simulink model "SISO_To_Workspace_Animation"  (R2024a)
settings: Solver=VariableStepAuto  StartTime=0.0  StopTime=10.0  RelTol=1e-3
undefined symbols (not defined in the file or in its folder): DINT, slplc
settings Model: Creator=Jack Vranicar  LastModifiedBy=Jack Vranicar

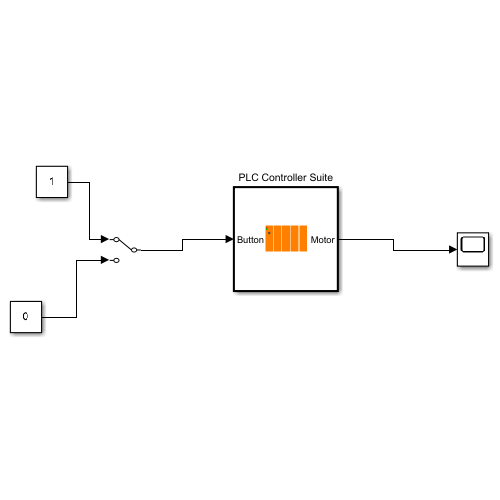
[thumbnail: Simulink's stored preview of the top-level diagram]
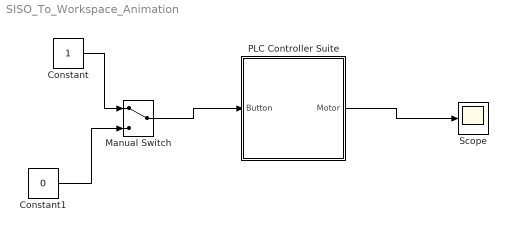
== system SISO_To_Workspace_Animation ==
  Constant : Constant  OutDataTypeStr=boolean
  Constant1 : Constant  Value=0  OutDataTypeStr=boolean
  Manual Switch : ManualSwitch
  PLC Controller Suite : Subsystem  TreatAsAtomicUnit=on  mask{PLCBlockType=PLCController, PLCPOUType=PLC Controller}
      mask init:
      | slplc.callbacks.initController(gcb);
      settings: OpenFcn=slplc.callbacks.openPOUBlock(gcb);
      mask Help: web([docroot '/plccoder/ref/plccontrollersuite' '.html']);
      mask DialogControl PLCBlockTitle Prompt: PLC Controller Block
  Scope : Scope
  wires:
  PLC Controller Suite/1(Motor) -> Scope/1
  Constant/1 -> Manual Switch/1
  Constant1/1 -> Manual Switch/2
  Manual Switch/1 -> PLC Controller Suite/1(Button)

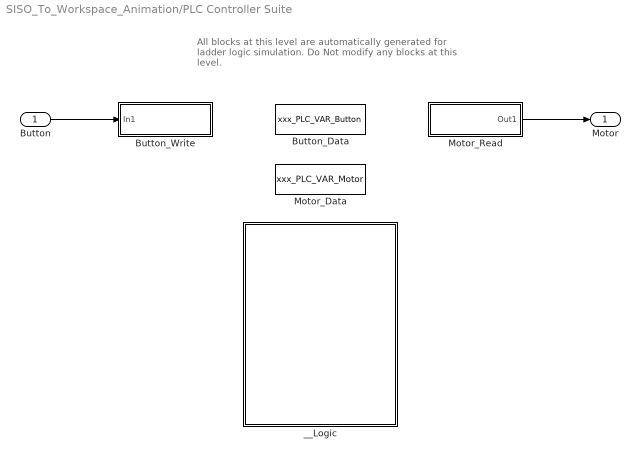
== system SISO_To_Workspace_Animation/PLC Controller Suite ==
  note: All blocks at this level are automatically generated for ladder logic simulation.
      | Do Not modify any blocks at this level.
  Button : Inport  OutDataTypeStr=boolean
  Button_Data : DataStoreMemory  Tag=POUVariable  Priority=10  DataStoreName=xxx_PLC_VAR_Button  ShowAdditionalParam=off  OutDataTypeStr=boolean  Dimensions=1
  Button_Write : Subsystem  Priority=11  DisableCoverage=on  TreatAsAtomicUnit=on  mask{PLCOperandTag=Button, PLCOperandExpression=xxx_PLC_VAR_Button, PLCBlockType=VarWrite, PLCPOUType=VarWrite}
      mask prompts: PLCOperandTag "Operand Tag:"
      mask init:
      | slplc.callbacks.initInstruction(gcb);
      mask Help: web([docroot '/plccoder/ref/varwrite' '.html']);
      mask DialogControl PLCBlockTitle Prompt: Variable Write
      mask Display: disp(get_param(gcb, 'PLCOperandTag'));
  Motor_Data : DataStoreMemory  Tag=POUVariable  Priority=10  DataStoreName=xxx_PLC_VAR_Motor  ShowAdditionalParam=off  OutDataTypeStr=boolean  Dimensions=1
  Motor_Read : Subsystem  Priority=13  DisableCoverage=on  TreatAsAtomicUnit=on  mask{PLCOperandTag=Motor, PLCOperandExpression=xxx_PLC_VAR_Motor, PLCBlockType=VarRead, PLCPOUType=VarRead}
      mask prompts: PLCOperandTag "Operand Tag"
      mask init:
      | block = gcb;
      | maskObj = Simulink.Mask.get(block);
      | maskObj.Display = sprintf('disp(''%s'');', PLCOperandTag);
      | slplc.callbacks.initInstruction(gcb);
      mask Help: web([docroot '/plccoder/ref/varread' '.html']);
      mask DialogControl PLCBlockTitle Prompt: Variable Read
      mask Display: disp('Motor');
  __Logic : Subsystem  Priority=12  TreatAsAtomicUnit=on
  Motor : Outport
  wires:
  Button/1 -> Button_Write/1(In1)
  Motor_Read/1(Out1) -> Motor/1

== system SISO_To_Workspace_Animation/PLC Controller Suite/Button_Write ==
  In1 : Inport
  __CoreVarWrite : Subsystem  Tag=CoreVarWriteBlock  DisableCoverage=on  TreatAsAtomicUnit=on  mask{PLCBlockType=CoreVarWrite}
      mask init:
      | slplc.callbacks.initCoreVariable(gcb, 'write');
      mask DialogControl PLCBlockTitle Prompt: Core Variable Write
  wires:
  In1/1 -> __CoreVarWrite/1(u)

== system SISO_To_Workspace_Animation/PLC Controller Suite/Motor_Read ==
  __CoreVarRead : Subsystem  Tag=CoreVarReadBlock  DisableCoverage=on  TreatAsAtomicUnit=on  mask{PLCBlockType=CoreVarRead}
      mask init:
      | slplc.callbacks.initCoreVariable(gcb, 'read');
      mask DialogControl PLCBlockTitle Prompt: Core Variable Read
  Out1 : Outport  VectorParamsAs1DForOutWhenUnconnected=off
  wires:
  __CoreVarRead/1(y) -> Out1/1

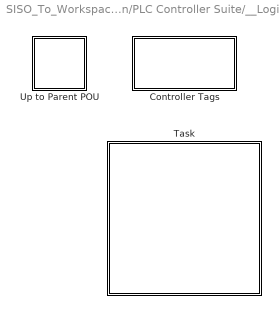
== system SISO_To_Workspace_Animation/PLC Controller Suite/__Logic ==
  Controller Tags : Subsystem  Tag=ControllerVariableSS  DisableCoverage=on  TreatAsAtomicUnit=on  mask{PLCVarButtonName=Button, PLCVarButtonAddress=<empty>, PLCVarButtonMapping=Input Symbol, PLCVarButtonPortIndex=1, PLCVarButtonDataType=boolean, PLCVarButtonSize=1, PLCVarButtonInitialValue=0, PLCVarButtonToDelete=off, PLCVarMotorName=Motor, PLCVarMotorAddress=<empty>, PLCVarMotorMapping=Output Symbol, PLCVarMotorPortIndex=1, PLCVarMotorDataType=boolean, PLCVarMotorSize=1, PLCVarMotorInitialValue=0, PLCVarMotorToDelete=off}
      mask init:
      | slplc.callbacks.initControllerVarSS(gcb);
      settings: OpenFcn=slplc.callbacks.openControllerVariableSS(gcb);
      mask Help: web([docroot '/plccoder/ref/controllertags' '.html']);
      mask TypeOptions PLCVarButtonMapping: Global Variable | Input Symbol | Output Symbol
      mask Callback PLCVarButtonMapping: slplc.callbacks.updateControllerVarSS(gcb);
      mask TypeOptions PLCVarButtonPortIndex: 1 | 2
      mask TypeOptions PLCVarMotorMapping: Global Variable | Input Symbol | Output Symbol
      mask Callback PLCVarMotorMapping: slplc.callbacks.updateControllerVarSS(gcb);
      mask TypeOptions PLCVarMotorPortIndex: 1 | 2
      mask DialogControl PLCBlockTitle Prompt: Global Variable and Symbol Spreadsheet
      mask DialogControl PLCVarListHeaderName Prompt: Name
      mask DialogControl PLCVarListHeaderAddress Prompt: Address (At)
      mask DialogControl PLCVarListHeaderMapping Prompt: Mapping Type
      mask DialogControl PLCVarListHeaderPortIndex Prompt: Port
      mask DialogControl PLCVarListHeaderDataType Prompt: Data Type
      mask DialogControl PLCVarListHeaderSize Prompt: Size
      mask DialogControl PLCVarListHeaderInitialValue Prompt: Initial Value
      mask DialogControl PLCVarListHeaderToDelete Prompt: Delete
  Task : Subsystem  TreatAsAtomicUnit=on  mask{PLCBlockType=Task, PLCPOUType=Task, PLCTaskWatchDog=0}
      settings: OpenFcn=slplc.callbacks.openTaskBlock(gcb);
      mask Help: web([docroot '/plccoder/ref/task' '.html']);
      mask DialogControl PLCBlockTitle Prompt: Task
  Up to Parent POU : Subsystem  DisableCoverage=on  TreatAsAtomicUnit=on  mask{PLCBlockType=OpenParentPOU}
      settings: OpenFcn=slplc.callbacks.openParentPOUBlock(gcb);
      mask Help: web([docroot '/plccoder/ref/uptoparentpou' '.html']);
      mask DialogControl PLCBlockTitle Prompt: Add Single Rung

== system SISO_To_Workspace_Animation/PLC Controller Suite/Button_Write/__CoreVarWrite ==
  u : Inport
  DataWrite : DataStoreWrite  DataStoreName=xxx_PLC_VAR_Button  IndexOptions=Index vector (dialog)  Indices=1  OutputSizes=1
  wires:
  u/1 -> DataWrite/1

== system SISO_To_Workspace_Animation/PLC Controller Suite/Motor_Read/__CoreVarRead ==
  DataRead : DataStoreRead  DataStoreName=xxx_PLC_VAR_Motor  IndexOptions=Index vector (dialog)  Indices=1  OutputSizes=1
  y : Outport  VectorParamsAs1DForOutWhenUnconnected=off
  wires:
  DataRead/1 -> y/1

== system SISO_To_Workspace_Animation/PLC Controller Suite/__Logic/Controller Tags ==

== system SISO_To_Workspace_Animation/PLC Controller Suite/__Logic/Task ==
  Program : Subsystem  TreatAsAtomicUnit=on  mask{PLCPOUType=Program, PLCPOULanguage=LD, PLCBlockType=LDProgram}
      mask prompts: PLCPOUType "POU Type:"
      mask init:
      | slplc.callbacks.initProgram(gcb);
      settings: OpenFcn=slplc.callbacks.openPOUBlock(gcb);
      mask Help: web([docroot '/plccoder/ref/ldprogram' '.html']);
      mask DialogControl PLCBlockTitle Prompt: Program
      mask DialogControl PLCEditPOU Prompt: Edit POU
      mask DialogControl PLCEditInterface Prompt: Edit Variables
  Up to Parent POU : Subsystem  DisableCoverage=on  TreatAsAtomicUnit=on  mask{PLCBlockType=OpenParentPOU}
      settings: OpenFcn=slplc.callbacks.openParentPOUBlock(gcb);
      mask Help: web([docroot '/plccoder/ref/uptoparentpou' '.html']);
      mask DialogControl PLCBlockTitle Prompt: Add Single Rung

== system SISO_To_Workspace_Animation/PLC Controller Suite/__Logic/Up to Parent POU ==

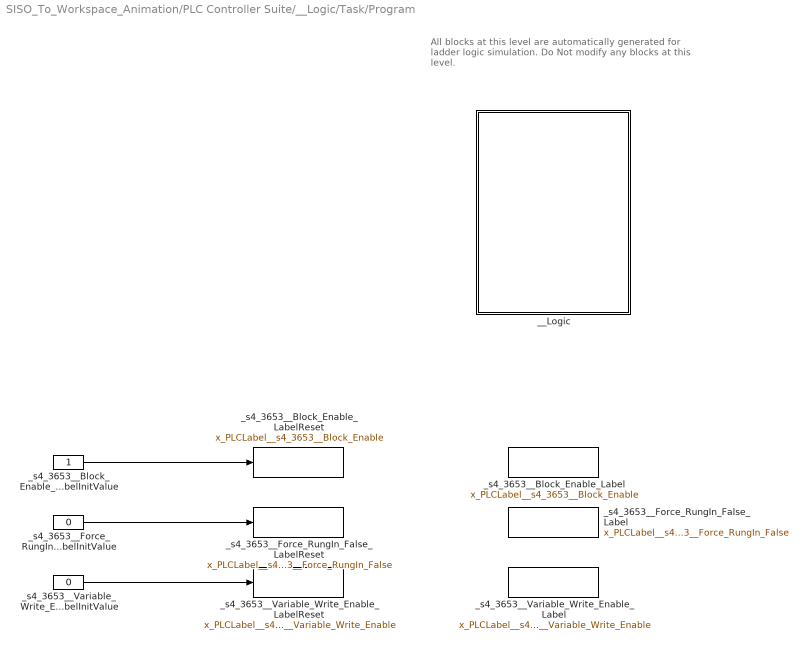
== system SISO_To_Workspace_Animation/PLC Controller Suite/__Logic/Task/Program ==
  note: All blocks at this level are automatically generated for ladder logic simulation.
      | Do Not modify any blocks at this level.
  __Logic : Subsystem  Priority=12  TreatAsAtomicUnit=on
  _s4_3653__Block_Enable_Label : DataStoreMemory  Priority=10  DataStoreName=x_PLCLabel__s4_3653__Block_Enable  InitialValue=1  ShowAdditionalParam=off  OutDataTypeStr=BOOL  Dimensions=1
  _s4_3653__Block_Enable_LabelInitValue : Constant  OutDataTypeStr=BOOL
  _s4_3653__Block_Enable_LabelReset : DataStoreWrite  Priority=11  DataStoreName=x_PLCLabel__s4_3653__Block_Enable  IndexOptions=Index vector (dialog)  Indices=1  OutputSizes=1
  _s4_3653__Force_RungIn_False_Label : DataStoreMemory  Priority=10  DataStoreName=x_PLCLabel__s4_3653__Force_RungIn_False  ShowAdditionalParam=off  OutDataTypeStr=BOOL  Dimensions=1
  _s4_3653__Force_RungIn_False_LabelInitValue : Constant  Value=0  OutDataTypeStr=BOOL
  _s4_3653__Force_RungIn_False_LabelReset : DataStoreWrite  Priority=11  DataStoreName=x_PLCLabel__s4_3653__Force_RungIn_False  IndexOptions=Index vector (dialog)  Indices=1  OutputSizes=1
  _s4_3653__Variable_Write_Enable_Label : DataStoreMemory  Priority=10  DataStoreName=x_PLCLabel__s4_3653__Variable_Write_Enable  ShowAdditionalParam=off  OutDataTypeStr=BOOL  Dimensions=1
  _s4_3653__Variable_Write_Enable_LabelInitValue : Constant  Value=0  OutDataTypeStr=BOOL
  _s4_3653__Variable_Write_Enable_LabelReset : DataStoreWrite  Priority=11  DataStoreName=x_PLCLabel__s4_3653__Variable_Write_Enable  IndexOptions=Index vector (dialog)  Indices=1  OutputSizes=1
  wires:
  _s4_3653__Block_Enable_LabelInitValue/1 -> _s4_3653__Block_Enable_LabelReset/1
  _s4_3653__Variable_Write_Enable_LabelInitValue/1 -> _s4_3653__Variable_Write_Enable_LabelReset/1
  _s4_3653__Force_RungIn_False_LabelInitValue/1 -> _s4_3653__Force_RungIn_False_LabelReset/1

== system SISO_To_Workspace_Animation/PLC Controller Suite/__Logic/Task/Up to Parent POU ==

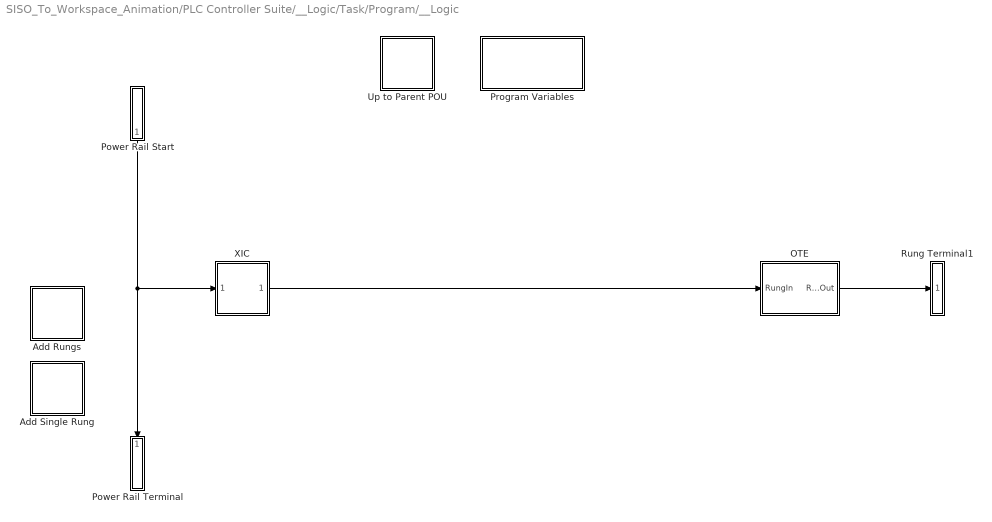
== system SISO_To_Workspace_Animation/PLC Controller Suite/__Logic/Task/Program/__Logic ==
  Add Rungs : Subsystem  DisableCoverage=on  TreatAsAtomicUnit=on  mask{PLCRungNumberToAdd=2, PLCBlockType=AddRungs}
      mask prompts: PLCRungNumberToAdd "Rung Number:"
      mask Help: web([docroot '/plccoder/ref/addrungs' '.html']);
      mask DialogControl PLCAddRungs Prompt: Add Rungs
      mask DialogControl PLCRungAddButton Prompt: Add
      mask DialogControl PLCRungAddButton Callback: slplc.callbacks.addLadderRungs(gcb);
      mask Display: disp(sprintf(['Add' newline 'Rungs']));
  Add Single Rung : Subsystem  DisableCoverage=on  TreatAsAtomicUnit=on  mask{PLCRungNumberToAdd=1, PLCBlockType=AddSingleRung}
      settings: OpenFcn=slplc.callbacks.addLadderRungs(gcb);
      mask Help: web([docroot '/plccoder/ref/addsinglerung' '.html']);
      mask DialogControl PLCAddRung Prompt: Add Single Rung
      mask Display: disp(sprintf(['Add' newline '1 Rung']));
  OTE : Subsystem  Priority=3  TreatAsAtomicUnit=on  mask{PLCOperandTag=Motor, PLCBlockType=OTE, PLCPOUType=Coil, PLCOperandExpression=xxx_PLC_VAR_Motor}
      mask prompts: PLCOperandTag "Operand Tag:"
      mask init:
      | slplc.callbacks.initInstruction(gcb);
      settings: AttributesFormatString=%<PLCOperandTag>
      mask Help: web([docroot '/plccoder/ref/ote' '.html']);
      mask DialogControl PLCBlockTitle Prompt: Output Energize (OTE)
  Power Rail Start : Subsystem  Priority=1  DisableCoverage=on  TreatAsAtomicUnit=on  mask{PLCBlockType=PowerRailStart}
      mask Help: web([docroot '/plccoder/ref/powerrailstart' '.html']);
      mask DialogControl PLCBlockTitle Prompt: Power Rail Start
      mask DialogControl PLCBlockDesc Prompt: This is the ladder diagram left power rail start block.
  Power Rail Terminal : Subsystem  DisableCoverage=on  TreatAsAtomicUnit=on  mask{PLCBlockType=PowerRailTerminal}
      mask Help: web([docroot '/plccoder/ref/powerrailterminal' '.html']);
      mask DialogControl PLCBlockTitle Prompt: Power Rail Terminal
      mask DialogControl PLCBlockDesc Prompt: This is the ladder diagram left power rail terminal block.
  Program Variables : Subsystem  Tag=ProgramVariableSS  DisableCoverage=on  TreatAsAtomicUnit=on  mask{PLCVarButtonName=Button, PLCVarButtonScope=External, PLCVarButtonPortType=Hidden, PLCVarButtonPortIndex=2, PLCVarButtonDataType=DINT, PLCVarButtonSize=-1, PLCVarButtonInitialValue=0, PLCVarButtonToDelete=off, PLCVarMotorName=Motor, PLCVarMotorScope=External, PLCVarMotorPortType=Hidden, PLCVarMotorPortIndex=2, PLCVarMotorDataType=DINT, PLCVarMotorSize=-1, PLCVarMotorInitialValue=0, PLCVarMotorToDelete=off}
      mask init:
      | slplc.callbacks.initPOUVarSS(gcb);
      settings: OpenFcn=slplc.callbacks.openProgramVariableSS(gcb);
      mask Help: web([docroot '/plccoder/ref/programvariables' '.html']);
      mask TypeOptions PLCVarButtonScope: Local | External
      mask Callback PLCVarButtonScope: slplc.callbacks.updatePOUVarSS(gcb);
      mask TypeOptions PLCVarButtonPortType: Hidden | Inport | Outport
      mask Callback PLCVarButtonPortType: slplc.callbacks.updatePOUVarSS(gcb);
      mask TypeOptions PLCVarButtonPortIndex: 1 | 2
      mask TypeOptions PLCVarMotorScope: Local | External
      mask Callback PLCVarMotorScope: slplc.callbacks.updatePOUVarSS(gcb);
      mask TypeOptions PLCVarMotorPortType: Hidden | Inport | Outport
      mask Callback PLCVarMotorPortType: slplc.callbacks.updatePOUVarSS(gcb);
      mask TypeOptions PLCVarMotorPortIndex: 1 | 2
      mask DialogControl PLCBlockTitle Prompt: Program Variable Spreadsheet
      mask DialogControl PLCVarListHeaderName Prompt: Name
      mask DialogControl PLCVarListHeaderScope Prompt: Scope
      mask DialogControl PLCVarListHeaderDataType Prompt: Data Type
      mask DialogControl PLCVarListHeaderSize Prompt: Size
      mask DialogControl PLCVarListHeaderInitialValue Prompt: Initial Value
      mask DialogControl PLCVarListHeaderToDelete Prompt: Delete
  Rung Terminal1 : Subsystem  Priority=4  DisableCoverage=on  TreatAsAtomicUnit=on  mask{PLCRungTerminalIndex=1, PLCBlockType=RungTerminal}
      settings: AttributesFormatString=Rung %<PLCRungTerminalIndex>
      mask Help: web([docroot '/plccoder/ref/rungterminal' '.html']);
      mask DialogControl PLCBlockTitle Prompt: Rung Terminal
      mask DialogControl PLCBlockDescText Prompt: This is the ladder diagram rung terminal.
  Up to Parent POU : Subsystem  DisableCoverage=on  TreatAsAtomicUnit=on  mask{PLCBlockType=OpenParentPOU}
      settings: OpenFcn=slplc.callbacks.openParentPOUBlock(gcb);
      mask Help: web([docroot '/plccoder/ref/uptoparentpou' '.html']);
      mask DialogControl PLCBlockTitle Prompt: Add Single Rung
  XIC : Subsystem  Priority=2  TreatAsAtomicUnit=on  mask{PLCOperandTag=Button, PLCBlockType=XIC, PLCPOUType=Contact, PLCOperandExpression=xxx_PLC_VAR_Button}
      mask prompts: PLCOperandTag "Operand Tag:"
      mask init:
      | slplc.callbacks.initInstruction(gcb);
      settings: AttributesFormatString=%<PLCOperandTag>
      mask Help: web([docroot '/plccoder/ref/xic' '.html']);
      mask DialogControl PLCBlockTitle Prompt: Examine If Closed (XIC)
  wires:
  Power Rail Start/1(PowerOut) -> Power Rail Terminal/1(PowerIn), XIC/1(RungIn)
  XIC/1(RungOut) -> OTE/1(RungIn)
  OTE/1(RungOut) -> Rung Terminal1/1(RungIn)

== system SISO_To_Workspace_Animation/PLC Controller Suite/__Logic/Task/Program/__Logic/Add Rungs ==

== system SISO_To_Workspace_Animation/PLC Controller Suite/__Logic/Task/Program/__Logic/Add Single Rung ==

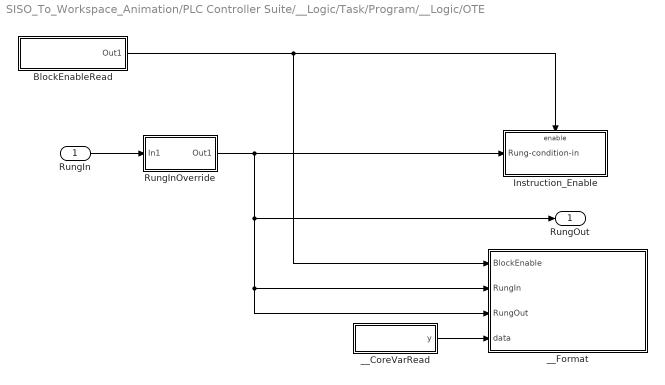
== system SISO_To_Workspace_Animation/PLC Controller Suite/__Logic/Task/Program/__Logic/OTE ==
  RungIn : Inport  PortDimensions=1
  BlockEnableRead : Subsystem  DisableCoverage=on  TreatAsAtomicUnit=on  mask{PLCLabelTag=_Block_Enable, PLCBlockType=BlockEnableRead}
      mask prompts: PLCLabelTag "Label Tag:"
      mask init:
      | block = gcb;
      | maskObj = Simulink.Mask.get(block);
      | maskObj.Display = sprintf('disp(''%s'');', PLCLabelTag);
      mask Help: web([docroot '/plccoder/ref/blockenableread' '.html']);
      mask DialogControl PLCBlockTitle Prompt: Block Enable Read
      mask Display: disp('_Block_Enable');
  Instruction_Enable : Subsystem  Priority=12  TreatAsAtomicUnit=on
  RungInOverride : Subsystem  DisableCoverage=on  TreatAsAtomicUnit=on
  __CoreVarRead : Subsystem  Tag=CoreVarReadBlock  DisableCoverage=on  TreatAsAtomicUnit=on  mask{PLCBlockType=CoreVarRead}
      mask init:
      | slplc.callbacks.initCoreVariable(gcb, 'read');
      mask Help: web([docroot '/plccoder/ref/__corevarread' '.html']);
      mask DialogControl PLCBlockTitle Prompt: Core Variable Read
  __Format : MATLAB Function  Tag=PLC_Format_Boolean  Priority=20  DisableCoverage=on  InitFcn=slplc.utils.setBlockAppearance('reset', '%<PLCOperandTag>');  StopFcn=slplc.utils.setBlockAppearance('reset', '%<PLCOperandTag>');  TreatAsAtomicUnit=on
  RungOut : Outport  OutDataTypeStr=BOOL  PortDimensions=1  InitialOutput=false  VectorParamsAs1DForOutWhenUnconnected=off
  wires:
  RungIn/1 -> RungInOverride/1(In1)
  BlockEnableRead/1(Out1) -> __Format/1(BlockEnable), Instruction_Enable/Enable
  RungInOverride/1(Out1) -> __Format/2(RungIn), __Format/3(RungOut), RungOut/1, Instruction_Enable/1(Rung-condition-in)
  __CoreVarRead/1(y) -> __Format/4(data)

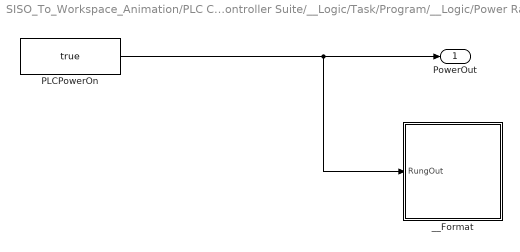
== system SISO_To_Workspace_Animation/PLC Controller Suite/__Logic/Task/Program/__Logic/Power Rail Start ==
  PLCPowerOn : Constant  Value=true  OutDataTypeStr=BOOL
  __Format : MATLAB Function  Tag=PLC_Format_ENO  Priority=20  DisableCoverage=on  InitFcn=slplc.utils.setBlockAppearance('reset', '', {'black', 'black'});  StopFcn=slplc.utils.setBlockAppearance('reset', '', {'black', 'black'});  TreatAsAtomicUnit=on
  PowerOut : Outport  VectorParamsAs1DForOutWhenUnconnected=off
  wires:
  PLCPowerOn/1 -> __Format/1(RungOut), PowerOut/1

== system SISO_To_Workspace_Animation/PLC Controller Suite/__Logic/Task/Program/__Logic/Power Rail Terminal ==
  PowerIn : Inport
  Terminator3 : Terminator
  wires:
  PowerIn/1 -> Terminator3/1

== system SISO_To_Workspace_Animation/PLC Controller Suite/__Logic/Task/Program/__Logic/Program Variables ==

== system SISO_To_Workspace_Animation/PLC Controller Suite/__Logic/Task/Program/__Logic/Rung Terminal1 ==
  RungIn : Inport
  Terminator : Terminator
  wires:
  RungIn/1 -> Terminator/1

== system SISO_To_Workspace_Animation/PLC Controller Suite/__Logic/Task/Program/__Logic/Up to Parent POU ==

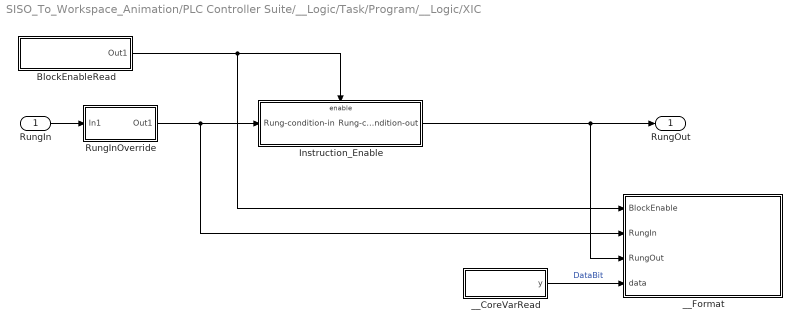
== system SISO_To_Workspace_Animation/PLC Controller Suite/__Logic/Task/Program/__Logic/XIC ==
  RungIn : Inport  PortDimensions=1
  BlockEnableRead : Subsystem  DisableCoverage=on  TreatAsAtomicUnit=on  mask{PLCLabelTag=_Block_Enable, PLCBlockType=BlockEnableRead}
      mask prompts: PLCLabelTag "Label Tag:"
      mask init:
      | block = gcb;
      | maskObj = Simulink.Mask.get(block);
      | maskObj.Display = sprintf('disp(''%s'');', PLCLabelTag);
      mask Help: web([docroot '/plccoder/ref/blockenableread' '.html']);
      mask DialogControl PLCBlockTitle Prompt: Block Enable Read
      mask Display: disp('_Block_Enable');
  Instruction_Enable : Subsystem  Priority=12  TreatAsAtomicUnit=on
  RungInOverride : Subsystem  DisableCoverage=on  TreatAsAtomicUnit=on
  __CoreVarRead : Subsystem  Tag=CoreVarReadBlock  DisableCoverage=on  TreatAsAtomicUnit=on  mask{PLCBlockType=CoreVarRead}
      mask init:
      | slplc.callbacks.initCoreVariable(gcb, 'read');
      mask Help: web([docroot '/plccoder/ref/__corevarread' '.html']);
      mask DialogControl PLCBlockTitle Prompt: Core Variable Read
  __Format : MATLAB Function  Tag=PLC_Format_Boolean  Priority=20  DisableCoverage=on  InitFcn=slplc.utils.setBlockAppearance('reset', '%<PLCOperandTag>');  StopFcn=slplc.utils.setBlockAppearance('reset', '%<PLCOperandTag>');  TreatAsAtomicUnit=on
  RungOut : Outport  OutDataTypeStr=BOOL  PortDimensions=1  InitialOutput=false  VectorParamsAs1DForOutWhenUnconnected=off
  wires:
  __CoreVarRead/1(y) -> __Format/4(data)  "DataBit"
  RungInOverride/1(Out1) -> Instruction_Enable/1(Rung-condition-in), __Format/2(RungIn)
  BlockEnableRead/1(Out1) -> Instruction_Enable/Enable, __Format/1(BlockEnable)
  Instruction_Enable/1(Rung-condition-out) -> RungOut/1, __Format/3(RungOut)
  RungIn/1 -> RungInOverride/1(In1)

== system SISO_To_Workspace_Animation/PLC Controller Suite/__Logic/Task/Program/__Logic/OTE/BlockEnableRead ==
  __CoreLabelRead : Subsystem  Tag=CoreVarReadBlock  DisableCoverage=on  TreatAsAtomicUnit=on  mask{PLCBlockType=CoreLabelRead}
      mask init:
      | slplc.callbacks.initRoutineLabelRead(gcb);
      mask Help: web([docroot '/plccoder/ref/__corelabelread' '.html']);
      mask DialogControl PLCBlockTitle Prompt: Core Label Read
  Out1 : Outport  VectorParamsAs1DForOutWhenUnconnected=off
  wires:
  __CoreLabelRead/1(Out1) -> Out1/1

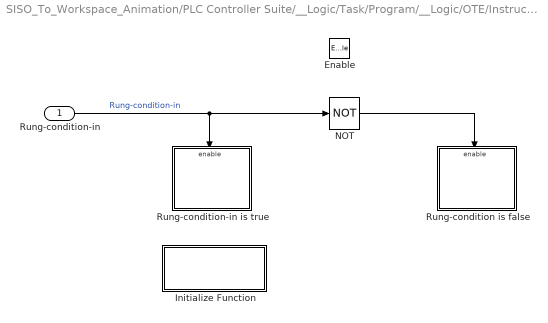
== system SISO_To_Workspace_Animation/PLC Controller Suite/__Logic/Task/Program/__Logic/OTE/Instruction_Enable ==
  Rung-condition-in : Inport  OutDataTypeStr=BOOL
  Enable : EnablePort
  Initialize Function : Subsystem  TreatAsAtomicUnit=on
  NOT : Logic  Operator=NOT  IconShape=distinctive  AllPortsSameDT=off  OutDataTypeStr=boolean
  Rung-condition is false : Subsystem  Priority=12  DisableCoverage=on
  Rung-condition-in is true : Subsystem  Priority=12  DisableCoverage=on
  wires:
  NOT/1 -> Rung-condition is false/Enable
  Rung-condition-in/1 -> Rung-condition-in is true/Enable, NOT/1  "Rung-condition-in"

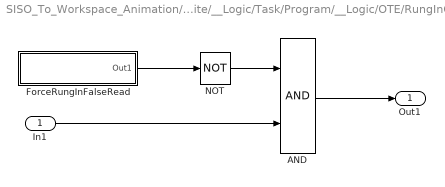
== system SISO_To_Workspace_Animation/PLC Controller Suite/__Logic/Task/Program/__Logic/OTE/RungInOverride ==
  In1 : Inport
  AND : Logic  AllPortsSameDT=off  OutDataTypeStr=boolean
  ForceRungInFalseRead : Subsystem  DisableCoverage=on  TreatAsAtomicUnit=on  mask{PLCLabelTag=_Force_RungIn_False, PLCBlockType=ForceRungInFalseRead}
      mask prompts: PLCLabelTag "Label Tag:"
      mask init:
      | block = gcb;
      | maskObj = Simulink.Mask.get(block);
      | maskObj.Display = sprintf('disp(''%s'');', PLCLabelTag);
      mask Help: web([docroot '/plccoder/ref/forcerunginfalseread' '.html']);
      mask DialogControl PLCBlockTitle Prompt: Force Rung-In False Read
      mask Display: disp('_Force_RungIn_False');
  NOT : Logic  Operator=NOT  IconShape=distinctive  AllPortsSameDT=off  OutDataTypeStr=boolean
  Out1 : Outport  VectorParamsAs1DForOutWhenUnconnected=off
  wires:
  AND/1 -> Out1/1
  In1/1 -> AND/2
  ForceRungInFalseRead/1(Out1) -> NOT/1
  NOT/1 -> AND/1

== system SISO_To_Workspace_Animation/PLC Controller Suite/__Logic/Task/Program/__Logic/OTE/__CoreVarRead ==
  DataRead : DataStoreRead  DataStoreName=xxx_PLC_VAR_Motor  IndexOptions=Index vector (dialog)  Indices=1  OutputSizes=1
  y : Outport  VectorParamsAs1DForOutWhenUnconnected=off
  wires:
  DataRead/1 -> y/1

== system SISO_To_Workspace_Animation/PLC Controller Suite/__Logic/Task/Program/__Logic/XIC/BlockEnableRead ==
  __CoreLabelRead : Subsystem  Tag=CoreVarReadBlock  DisableCoverage=on  TreatAsAtomicUnit=on  mask{PLCBlockType=CoreLabelRead}
      mask init:
      | slplc.callbacks.initRoutineLabelRead(gcb);
      mask Help: web([docroot '/plccoder/ref/__corelabelread' '.html']);
      mask DialogControl PLCBlockTitle Prompt: Core Label Read
  Out1 : Outport  VectorParamsAs1DForOutWhenUnconnected=off
  wires:
  __CoreLabelRead/1(Out1) -> Out1/1

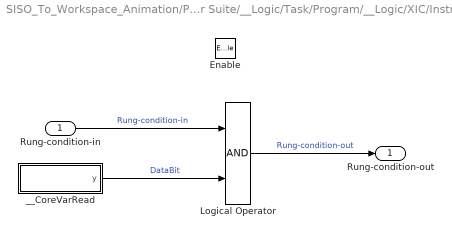
== system SISO_To_Workspace_Animation/PLC Controller Suite/__Logic/Task/Program/__Logic/XIC/Instruction_Enable ==
  Rung-condition-in : Inport  OutDataTypeStr=BOOL
  Enable : EnablePort
  Logical Operator : Logic  OutDataTypeStr=BOOL
  __CoreVarRead : Subsystem  Tag=CoreVarReadBlock  DisableCoverage=on  TreatAsAtomicUnit=on  mask{PLCBlockType=CoreVarRead}
      mask init:
      | slplc.callbacks.initCoreVariable(gcb, 'read');
      mask Help: web([docroot '/plccoder/ref/__corevarread' '.html']);
      mask DialogControl PLCBlockTitle Prompt: Core Variable Read
  Rung-condition-out : Outport  VectorParamsAs1DForOutWhenUnconnected=off
  wires:
  Rung-condition-in/1 -> Logical Operator/1  "Rung-condition-in"
  Logical Operator/1 -> Rung-condition-out/1  "Rung-condition-out"
  __CoreVarRead/1(y) -> Logical Operator/2  "DataBit"

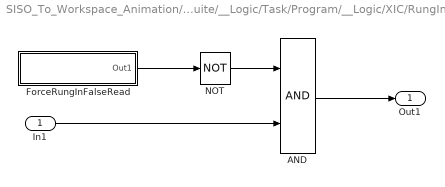
== system SISO_To_Workspace_Animation/PLC Controller Suite/__Logic/Task/Program/__Logic/XIC/RungInOverride ==
  In1 : Inport
  AND : Logic  AllPortsSameDT=off  OutDataTypeStr=boolean
  ForceRungInFalseRead : Subsystem  DisableCoverage=on  TreatAsAtomicUnit=on  mask{PLCLabelTag=_Force_RungIn_False, PLCBlockType=ForceRungInFalseRead}
      mask prompts: PLCLabelTag "Label Tag:"
      mask init:
      | block = gcb;
      | maskObj = Simulink.Mask.get(block);
      | maskObj.Display = sprintf('disp(''%s'');', PLCLabelTag);
      mask Help: web([docroot '/plccoder/ref/forcerunginfalseread' '.html']);
      mask DialogControl PLCBlockTitle Prompt: Force Rung-In False Read
      mask Display: disp('_Force_RungIn_False');
  NOT : Logic  Operator=NOT  IconShape=distinctive  AllPortsSameDT=off  OutDataTypeStr=boolean
  Out1 : Outport  VectorParamsAs1DForOutWhenUnconnected=off
  wires:
  AND/1 -> Out1/1
  In1/1 -> AND/2
  ForceRungInFalseRead/1(Out1) -> NOT/1
  NOT/1 -> AND/1

== system SISO_To_Workspace_Animation/PLC Controller Suite/__Logic/Task/Program/__Logic/XIC/__CoreVarRead ==
  DataRead : DataStoreRead  DataStoreName=xxx_PLC_VAR_Button  IndexOptions=Index vector (dialog)  Indices=1  OutputSizes=1
  y : Outport  VectorParamsAs1DForOutWhenUnconnected=off
  wires:
  DataRead/1 -> y/1

== system SISO_To_Workspace_Animation/PLC Controller Suite/__Logic/Task/Program/__Logic/OTE/BlockEnableRead/__CoreLabelRead ==
  DataRead : DataStoreRead  DataStoreName=x_PLCLabel__s4_3653__Block_Enable  IndexOptions=Index vector (dialog)  Indices=1  OutputSizes=1
  Out1 : Outport  VectorParamsAs1DForOutWhenUnconnected=off
  wires:
  DataRead/1 -> Out1/1

== system SISO_To_Workspace_Animation/PLC Controller Suite/__Logic/Task/Program/__Logic/OTE/Instruction_Enable/Initialize Function ==
  Constant : Constant  Value=0  OutDataTypeStr=BOOL
  Event Listener : EventListener  DisableCoverage=on  EventName=reset
  __CoreVarWrite : Subsystem  Tag=CoreVarWriteBlock  DisableCoverage=on  TreatAsAtomicUnit=on  mask{PLCBlockType=CoreVarWrite}
      mask init:
      | slplc.callbacks.initCoreVariable(gcb, 'write');
      mask Help: web([docroot '/plccoder/ref/__corevarwrite' '.html']);
      mask DialogControl PLCBlockTitle Prompt: Core Variable Write
  wires:
  Constant/1 -> __CoreVarWrite/1(u)

== system SISO_To_Workspace_Animation/PLC Controller Suite/__Logic/Task/Program/__Logic/OTE/Instruction_Enable/Rung-condition is false ==
  Enable : EnablePort
  Constant : Constant  Value=0  OutDataTypeStr=BOOL
  __CoreVarWrite : Subsystem  Tag=CoreVarWriteBlock  DisableCoverage=on  TreatAsAtomicUnit=on  mask{PLCBlockType=CoreVarWrite}
      mask init:
      | slplc.callbacks.initCoreVariable(gcb, 'write');
      mask Help: web([docroot '/plccoder/ref/__corevarwrite' '.html']);
      mask DialogControl PLCBlockTitle Prompt: Core Variable Write
  wires:
  Constant/1 -> __CoreVarWrite/1(u)

== system SISO_To_Workspace_Animation/PLC Controller Suite/__Logic/Task/Program/__Logic/OTE/Instruction_Enable/Rung-condition-in is true ==
  Enable : EnablePort
  Constant : Constant  OutDataTypeStr=BOOL
  __CoreVarWrite : Subsystem  Tag=CoreVarWriteBlock  DisableCoverage=on  TreatAsAtomicUnit=on  mask{PLCBlockType=CoreVarWrite}
      mask init:
      | slplc.callbacks.initCoreVariable(gcb, 'write');
      mask Help: web([docroot '/plccoder/ref/__corevarwrite' '.html']);
      mask DialogControl PLCBlockTitle Prompt: Core Variable Write
  wires:
  Constant/1 -> __CoreVarWrite/1(u)

== system SISO_To_Workspace_Animation/PLC Controller Suite/__Logic/Task/Program/__Logic/OTE/RungInOverride/ForceRungInFalseRead ==
  __CoreLabelRead : Subsystem  Tag=CoreVarReadBlock  DisableCoverage=on  TreatAsAtomicUnit=on  mask{PLCBlockType=CoreLabelRead}
      mask init:
      | slplc.callbacks.initRoutineLabelRead(gcb);
      mask Help: web([docroot '/plccoder/ref/__corelabelread' '.html']);
      mask DialogControl PLCBlockTitle Prompt: Core Label Read
  Out1 : Outport  VectorParamsAs1DForOutWhenUnconnected=off
  wires:
  __CoreLabelRead/1(Out1) -> Out1/1

== system SISO_To_Workspace_Animation/PLC Controller Suite/__Logic/Task/Program/__Logic/XIC/BlockEnableRead/__CoreLabelRead ==
  DataRead : DataStoreRead  DataStoreName=x_PLCLabel__s4_3653__Block_Enable  IndexOptions=Index vector (dialog)  Indices=1  OutputSizes=1
  Out1 : Outport  VectorParamsAs1DForOutWhenUnconnected=off
  wires:
  DataRead/1 -> Out1/1

== system SISO_To_Workspace_Animation/PLC Controller Suite/__Logic/Task/Program/__Logic/XIC/Instruction_Enable/__CoreVarRead ==
  DataRead : DataStoreRead  DataStoreName=xxx_PLC_VAR_Button  IndexOptions=Index vector (dialog)  Indices=1  OutputSizes=1
  y : Outport  VectorParamsAs1DForOutWhenUnconnected=off
  wires:
  DataRead/1 -> y/1

== system SISO_To_Workspace_Animation/PLC Controller Suite/__Logic/Task/Program/__Logic/XIC/RungInOverride/ForceRungInFalseRead ==
  __CoreLabelRead : Subsystem  Tag=CoreVarReadBlock  DisableCoverage=on  TreatAsAtomicUnit=on  mask{PLCBlockType=CoreLabelRead}
      mask init:
      | slplc.callbacks.initRoutineLabelRead(gcb);
      mask Help: web([docroot '/plccoder/ref/__corelabelread' '.html']);
      mask DialogControl PLCBlockTitle Prompt: Core Label Read
  Out1 : Outport  VectorParamsAs1DForOutWhenUnconnected=off
  wires:
  __CoreLabelRead/1(Out1) -> Out1/1

== system SISO_To_Workspace_Animation/PLC Controller Suite/__Logic/Task/Program/__Logic/OTE/Instruction_Enable/Initialize Function/__CoreVarWrite ==
  u : Inport
  DataWrite : DataStoreWrite  DataStoreName=xxx_PLC_VAR_Motor  IndexOptions=Index vector (dialog)  Indices=1  OutputSizes=1
  wires:
  u/1 -> DataWrite/1

== system SISO_To_Workspace_Animation/PLC Controller Suite/__Logic/Task/Program/__Logic/OTE/Instruction_Enable/Rung-condition is false/__CoreVarWrite ==
  u : Inport
  DataWrite : DataStoreWrite  DataStoreName=xxx_PLC_VAR_Motor  IndexOptions=Index vector (dialog)  Indices=1  OutputSizes=1
  wires:
  u/1 -> DataWrite/1

== system SISO_To_Workspace_Animation/PLC Controller Suite/__Logic/Task/Program/__Logic/OTE/Instruction_Enable/Rung-condition-in is true/__CoreVarWrite ==
  u : Inport
  DataWrite : DataStoreWrite  DataStoreName=xxx_PLC_VAR_Motor  IndexOptions=Index vector (dialog)  Indices=1  OutputSizes=1
  wires:
  u/1 -> DataWrite/1

== system SISO_To_Workspace_Animation/PLC Controller Suite/__Logic/Task/Program/__Logic/OTE/RungInOverride/ForceRungInFalseRead/__CoreLabelRead ==
  DataRead : DataStoreRead  DataStoreName=x_PLCLabel__s4_3653__Force_RungIn_False  IndexOptions=Index vector (dialog)  Indices=1  OutputSizes=1
  Out1 : Outport  VectorParamsAs1DForOutWhenUnconnected=off
  wires:
  DataRead/1 -> Out1/1

== system SISO_To_Workspace_Animation/PLC Controller Suite/__Logic/Task/Program/__Logic/XIC/RungInOverride/ForceRungInFalseRead/__CoreLabelRead ==
  DataRead : DataStoreRead  DataStoreName=x_PLCLabel__s4_3653__Force_RungIn_False  IndexOptions=Index vector (dialog)  Indices=1  OutputSizes=1
  Out1 : Outport  VectorParamsAs1DForOutWhenUnconnected=off
  wires:
  DataRead/1 -> Out1/1

== matlab function SISO_To_Workspace_Animation/PLC Controller Suite/__Logic/Task/Program/__Logic/XIC/__Format ==
  data: BlockEnable input; RungIn input; RungOut input; data input
function setBlockFormat(BlockEnable, RungIn, RungOut, data)

if data~=0 && data~=1
    error('slplc:inivalidBooleanValue', 'Invalid boolean value %d', data);
end
data = logical(data);

% set parent block colors
coder.extrinsic('slplc.utils.setBlockAppearance');
persistent lastBlockEnable lastRungIn lastRungOut lastData isInit lastAnimation lastDataShow;
if isempty(lastBlockEnable)
    lastBlockEnable = true;
end
if isempty(lastRungIn)
    lastRungIn = false;
end
if isempty(lastRungOut)
    lastRungOut = false;
end
if isempty(lastData)
    lastData = data;
end
if isempty(isInit)
    isInit = true;
else
    isInit = false;
end
if isempty(lastAnimation)
    lastAnimation = false;
end
if isempty(lastDataShow)
    lastDataShow = false;
end

[animation, dataShow] = slplc.utils.setBlockAppearance('set', '%<PLCOperandTag>', {}, {}, ...
    ' = ', {'ForegroundColor'}, ...
    isInit,  ...
    BlockEnable, lastBlockEnable, ...
    RungIn,  lastRungIn, ...
    RungOut, lastRungOut, ...
    data, lastData, ...
    lastAnimation, lastDataShow);

lastBlockEnable = BlockEnable;
lastRungIn      = RungIn;
lastRungOut     = RungOut;
lastData        = data;
lastAnimation   = animation;
lastDataShow    = dataShow;
end

== matlab function SISO_To_Workspace_Animation/PLC Controller Suite/__Logic/Task/Program/__Logic/OTE/__Format ==
  data: BlockEnable input; RungIn input; RungOut input; data input
function setBlockFormat(BlockEnable, RungIn, RungOut, data)

if data~=0 && data~=1
    error('slplc:inivalidBooleanValue', 'Invalid boolean value %d', data);
end
data = logical(data);

% set parent block colors
coder.extrinsic('slplc.utils.setBlockAppearance');
persistent lastBlockEnable lastRungIn lastRungOut lastData isInit lastAnimation lastDataShow;
if isempty(lastBlockEnable)
    lastBlockEnable = true;
end
if isempty(lastRungIn)
    lastRungIn = false;
end
if isempty(lastRungOut)
    lastRungOut = false;
end
if isempty(lastData)
    lastData = data;
end
if isempty(isInit)
    isInit = true;
else
    isInit = false;
end
if isempty(lastAnimation)
    lastAnimation = false;
end
if isempty(lastDataShow)
    lastDataShow = false;
end

[animation, dataShow] = slplc.utils.setBlockAppearance('set', '%<PLCOperandTag>', {}, {}, ...
    ' = ', {'ForegroundColor'}, ...
    isInit,  ...
    BlockEnable, lastBlockEnable, ...
    RungIn,  lastRungIn, ...
    RungOut, lastRungOut, ...
    data, lastData, ...
    lastAnimation, lastDataShow);

lastBlockEnable = BlockEnable;
lastRungIn      = RungIn;
lastRungOut     = RungOut;
lastData        = data;
lastAnimation   = animation;
lastDataShow    = dataShow;
end

== matlab function SISO_To_Workspace_Animation/PLC Controller Suite/__Logic/Task/Program/__Logic/Power Rail Start/__Format ==
  data: RungOut input
function setBlockFormat(RungOut)
% set parent block colors
coder.extrinsic('slplc.utils.setBlockAppearance');
persistent isInit lastRungOut lastAnimation lastRungOutShow;

if isempty(isInit)
    isInit = true;
else
    isInit = false;
end

if isempty(lastRungOut)
    lastRungOut = RungOut;
end

if isempty(lastAnimation)
    lastAnimation = false;
end

if isempty(lastRungOutShow)
    lastRungOutShow = false;
end

[animation, dataShow] = slplc.utils.setBlockAppearance('set', '', {'black', 'black'}, {}, ...
    '', {'ForegroundColor', 'BackgroundColor'}, ...
    isInit,  ...
    true,  true, ...
    RungOut,   lastRungOut, ...
    RungOut,   lastRungOut, ...
    [],    [], ...
    lastAnimation, lastRungOutShow);

lastRungOut         = RungOut;
lastAnimation       = animation;
lastRungOutShow     = dataShow;
end
